simulink library "cntrl_atti_red_indi_lib"  (R2018b)
settings: Solver=VariableStepAuto  StartTime=0.0  StopTime=10.0  RelTol=1e-3
undefined symbols (not defined in the file or in its folder): atti_cntrl, DiscIntNeverNeededParam
libraries: angles_lib x3, ndi_lib x2, $bdroot x2, axes_transformation_lib x1
settings Model: Creator=Ybeyer  LastModifiedBy=Yannic
settings SFSimCC: SimUseLocalCustomCode=off
settings RTWCC: RTWUseLocalCustomCode=off
settings CodeAppCC: StateflowObjectComments=on

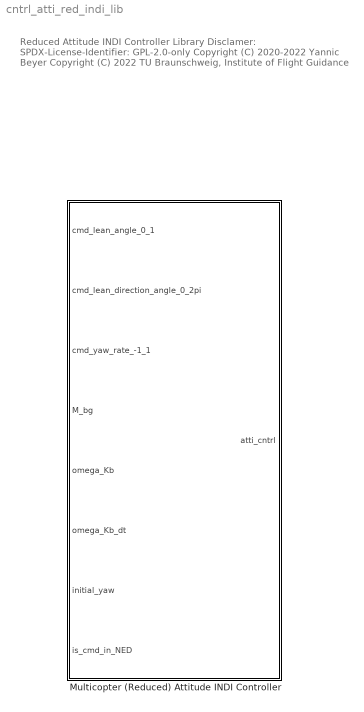
== system cntrl_atti_red_indi_lib ==
  note: Reduced Attitude INDI Controller Library
      |
      | Disclamer:
      | SPDX-License-Identifier: GPL-2.0-only
      |
      | Copyright (C) 2020-2022 Yannic Beyer
      | Copyright (C) 2022 TU Braunschweig, Institute of Flight Guidance
  Multicopter (Reduced) Attitude INDI Controller : Subsystem  mask{atti_cntrl=atti_cntrl, T=0.01}
      mask prompts: atti_cntrl "reduced attitude control struct"; T "inner loop time constant"
      mask Help: https://www.mathworks.com
      mask DialogControl DescGroupVar Prompt: INDI Reduced Attitude Controller
      mask DialogControl DescTextVar Prompt: To initialize the reduced attitude control struct see cntrlAttiRedIndiLoadParams

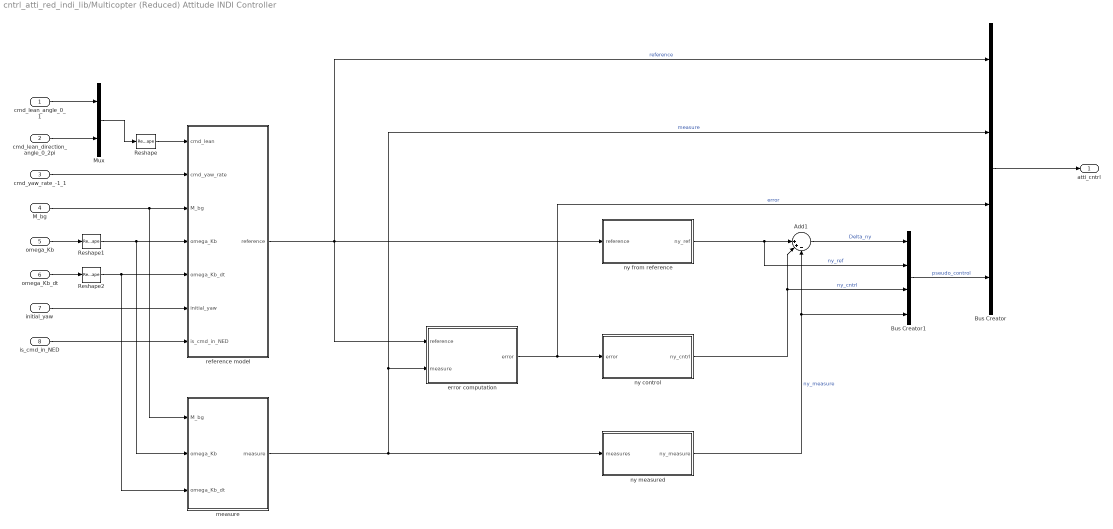
== system cntrl_atti_red_indi_lib/Multicopter (Reduced) Attitude INDI Controller ==
  cmd_lean_angle_0_1 : Inport
  cmd_lean_direction_angle_0_2pi : Inport  Port=2
  cmd_yaw_rate_-1_1 : Inport  Port=3
  M_bg : Inport  Port=4
  omega_Kb : Inport  Port=5
  omega_Kb_dt : Inport  Port=6
  initial_yaw : Inport  Port=7
  is_cmd_in_NED : Inport  Port=8
  Add1 : Sum  Inputs=||++-
  Bus Creator : BusCreator  Inputs=4
  Bus Creator1 : BusCreator  Inputs=4
  Mux : Mux  Inputs=2
  Reshape : Reshape  OutputDimensionality=Column vector (2-D)
  Reshape1 : Reshape  OutputDimensionality=Column vector (2-D)
  Reshape2 : Reshape  OutputDimensionality=Column vector (2-D)
  error computation : Subsystem
  measure : Subsystem
  ny control : Subsystem
  ny from reference : Subsystem
  ny measured : Subsystem
  reference model : Subsystem
  atti_cntrl : Outport
  wires:
  ny from reference/1(ny_ref) -> Bus Creator1/2, Add1/1  "ny_ref"
  Mux/1 -> Reshape/1
  error computation/1(error) -> ny control/1(error), Bus Creator/3  "error"
  omega_Kb_dt/1 -> Reshape2/1
  ny control/1(ny_cntrl) -> Bus Creator1/3, Add1/2  "ny_cntrl"
  ny measured/1(ny_measure) -> Bus Creator1/4, Add1/3  "ny_measure"
  reference model/1(reference) -> Bus Creator/1, error computation/1(reference), ny from reference/1(reference)  "reference"
  initial_yaw/1 -> reference model/6(initial_yaw)
  Bus Creator/1 -> atti_cntrl/1
  Bus Creator1/1 -> Bus Creator/4  "pseudo_control"
  Add1/1 -> Bus Creator1/1  "Delta_ny"
  M_bg/1 -> measure/1(M_bg), reference model/3(M_bg)
  omega_Kb/1 -> Reshape1/1
  measure/1(measure) -> Bus Creator/2, error computation/2(measure), ny measured/1(measures)  "measure"
  Reshape/1 -> reference model/1(cmd_lean)
  Reshape1/1 -> measure/2(omega_Kb), reference model/4(omega_Kb)
  Reshape2/1 -> measure/3(omega_Kb_dt), reference model/5(omega_Kb_dt)
  cmd_lean_angle_0_1/1 -> Mux/1
  cmd_lean_direction_angle_0_2pi/1 -> Mux/2
  cmd_yaw_rate_-1_1/1 -> reference model/2(cmd_yaw_rate)
  is_cmd_in_NED/1 -> reference model/7(is_cmd_in_NED)

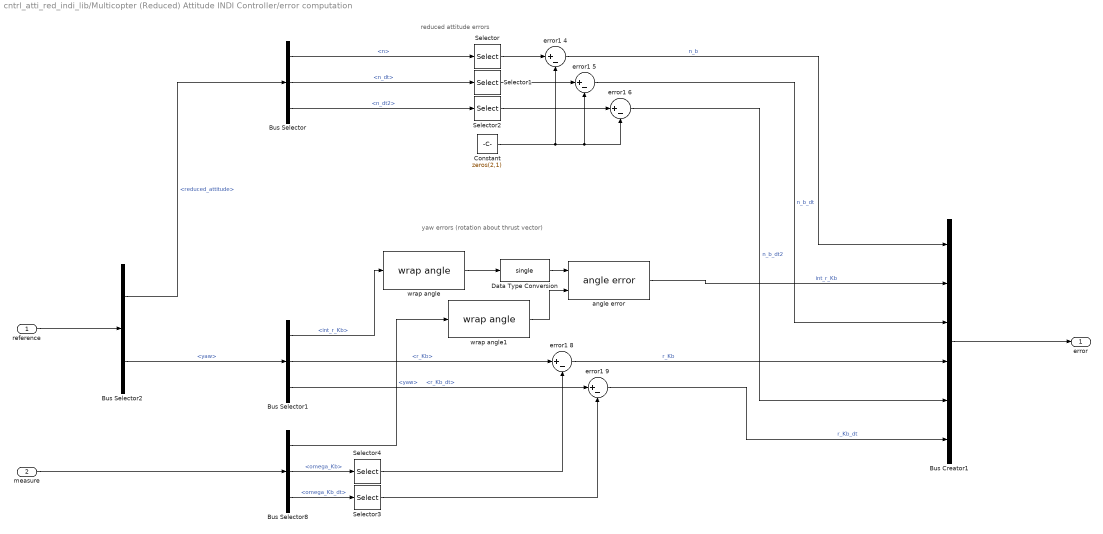
== system cntrl_atti_red_indi_lib/Multicopter (Reduced) Attitude INDI Controller/error computation ==
  note: reduced attitude errors
  note: yaw errors (rotation about thrust vector)
  reference : Inport
  measure : Inport  Port=2
  Bus Creator1 : BusCreator  Inputs=6
  Bus Selector : BusSelector  OutputSignals=n,n_dt,n_dt2
  Bus Selector1 : BusSelector  OutputSignals=int_r_Kb,r_Kb,r_Kb_dt
  Bus Selector2 : BusSelector  OutputSignals=reduced_attitude,yaw
  Bus Selector8 : BusSelector  OutputSignals=yaw,omega_Kb,omega_Kb_dt
  Constant : Constant  Value=zeros(2,1)  OutDataTypeStr=Inherit: Inherit via back propagation
  Data Type Conversion : DataTypeConversion  OutDataTypeStr=single
  Selector : Selector  InputPortWidth=3  IndexOptions=Index vector (dialog)  Indices=[1,2]  OutputSizes=1
  Selector1 : Selector  InputPortWidth=3  IndexOptions=Index vector (dialog)  Indices=[1,2]  OutputSizes=1
  Selector2 : Selector  InputPortWidth=3  IndexOptions=Index vector (dialog)  Indices=[1,2]  OutputSizes=1
  Selector3 : Selector  InputPortWidth=3  IndexOptions=Index vector (dialog)  Indices=3  OutputSizes=1
  Selector4 : Selector  InputPortWidth=3  IndexOptions=Index vector (dialog)  Indices=3  OutputSizes=1
  angle error : angles_lib/angle error  SystemSampleTime=-1
      settings: SourceProductName=LADAC
  error1 {4..6,8..9} (5 alike) : Sum  Inputs=|+-
  wrap angle : angles_lib/wrap angle  SystemSampleTime=-1
      settings: SourceProductName=LADAC
  wrap angle1 : angles_lib/wrap angle  SystemSampleTime=-1
      settings: SourceProductName=LADAC
  error : Outport
  wires:
  error1 4/1 -> Bus Creator1/1  "n_b"
  reference/1 -> Bus Selector2/1
  Bus Selector/1 -> Selector/1  "<n>"
  Bus Selector/2 -> Selector1/1  "<n_dt>"
  Bus Selector/3 -> Selector2/1  "<n_dt2>"
  Bus Selector2/1 -> Bus Selector/1  "<reduced_attitude>"
  Bus Creator1/1 -> error/1
  Selector/1 -> error1 4/1
  Selector1/1 -> error1 5/1
  Selector2/1 -> error1 6/1
  Constant/1 -> error1 6/2, error1 5/2, error1 4/2
  Bus Selector2/2 -> Bus Selector1/1  "<yaw>"
  Bus Selector1/1 -> wrap angle/1  "<int_r_Kb>"
  Bus Selector1/2 -> error1 8/1  "<r_Kb>"
  Bus Selector1/3 -> error1 9/1  "<r_Kb_dt>"
  measure/1 -> Bus Selector8/1
  Bus Selector8/3 -> Selector3/1  "<omega_Kb_dt>"
  Bus Selector8/2 -> Selector4/1  "<omega_Kb>"
  Bus Selector8/1 -> wrap angle1/1  "<yaw>"
  Selector4/1 -> error1 8/2
  Selector3/1 -> error1 9/2
  angle error/1 -> Bus Creator1/2  "int_r_Kb"
  error1 8/1 -> Bus Creator1/4  "r_Kb"
  error1 5/1 -> Bus Creator1/3  "n_b_dt"
  error1 6/1 -> Bus Creator1/5  "n_b_dt2"
  error1 9/1 -> Bus Creator1/6  "r_Kb_dt"
  wrap angle1/1 -> angle error/2
  wrap angle/1 -> Data Type Conversion/1
  Data Type Conversion/1 -> angle error/1

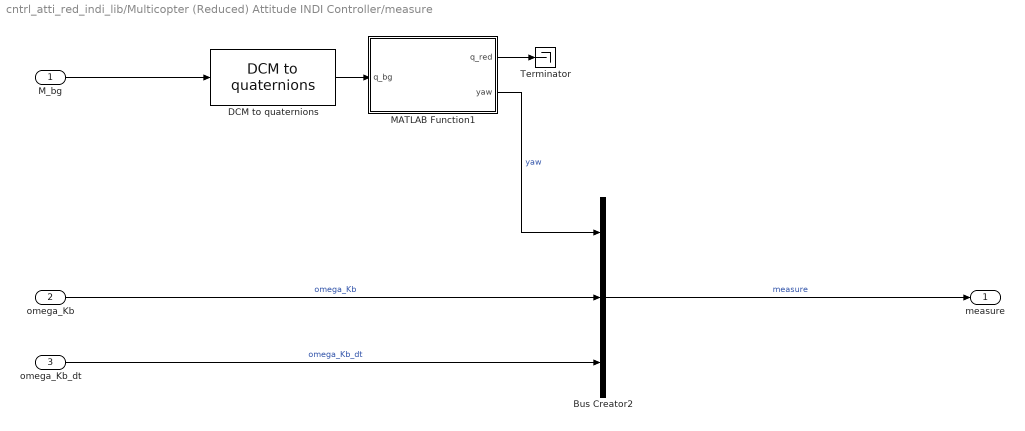
== system cntrl_atti_red_indi_lib/Multicopter (Reduced) Attitude INDI Controller/measure ==
  M_bg : Inport
  omega_Kb : Inport  Port=2
  omega_Kb_dt : Inport  Port=3
  Bus Creator2 : BusCreator  Inputs=3
  DCM to quaternions : axes_transformation_lib/DCM to quaternions  SystemSampleTime=-1
  MATLAB Function1 : MATLAB Function  TreatAsAtomicUnit=on
  Terminator : Terminator
  measure : Outport
  wires:
  DCM to quaternions/1 -> MATLAB Function1/1(q_bg)
  MATLAB Function1/1(q_red) -> Terminator/1
  MATLAB Function1/2(yaw) -> Bus Creator2/1  "yaw"
  M_bg/1 -> DCM to quaternions/1
  omega_Kb/1 -> Bus Creator2/2  "omega_Kb"
  omega_Kb_dt/1 -> Bus Creator2/3  "omega_Kb_dt"
  Bus Creator2/1 -> measure/1  "measure"

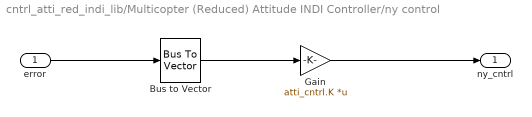
== system cntrl_atti_red_indi_lib/Multicopter (Reduced) Attitude INDI Controller/ny control ==
  error : Inport
  Bus to Vector : BusToVector
  Gain : Gain  Gain=atti_cntrl.K  Multiplication=Matrix(K*u)
  ny_cntrl : Outport
  wires:
  Gain/1 -> ny_cntrl/1
  error/1 -> Bus to Vector/1
  Bus to Vector/1 -> Gain/1

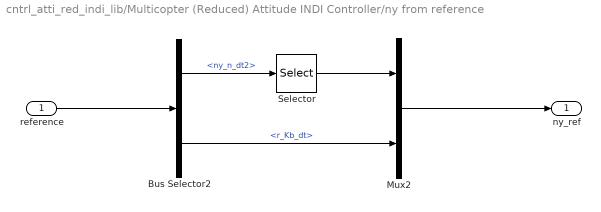
== system cntrl_atti_red_indi_lib/Multicopter (Reduced) Attitude INDI Controller/ny from reference ==
  reference : Inport
  Bus Selector2 : BusSelector  OutputSignals=reduced_attitude.ny_n_dt2,yaw.r_Kb_dt
  Mux2 : Mux  Inputs=2
  Selector : Selector  InputPortWidth=3  IndexOptions=Index vector (dialog)  Indices=[1,2]  OutputSizes=1
  ny_ref : Outport
  wires:
  reference/1 -> Bus Selector2/1
  Mux2/1 -> ny_ref/1
  Bus Selector2/2 -> Mux2/2  "<r_Kb_dt>"
  Bus Selector2/1 -> Selector/1  "<ny_n_dt2>"
  Selector/1 -> Mux2/1

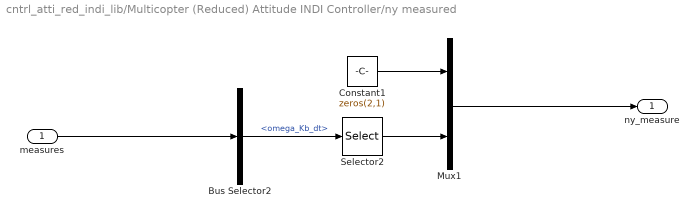
== system cntrl_atti_red_indi_lib/Multicopter (Reduced) Attitude INDI Controller/ny measured ==
  measures : Inport
  Bus Selector2 : BusSelector  OutputSignals=attitude.omega_Kb_dt
  Constant1 : Constant  Value=zeros(2,1)  OutDataTypeStr=Inherit: Inherit via back propagation
  Mux1 : Mux  Inputs=2
  Selector2 : Selector  InputPortWidth=3  IndexOptions=Index vector (dialog)  Indices=3  OutputSizes=1
  ny_measure : Outport
  wires:
  Bus Selector2/1 -> Selector2/1  "<omega_Kb_dt>"
  measures/1 -> Bus Selector2/1
  Mux1/1 -> ny_measure/1
  Selector2/1 -> Mux1/2
  Constant1/1 -> Mux1/1

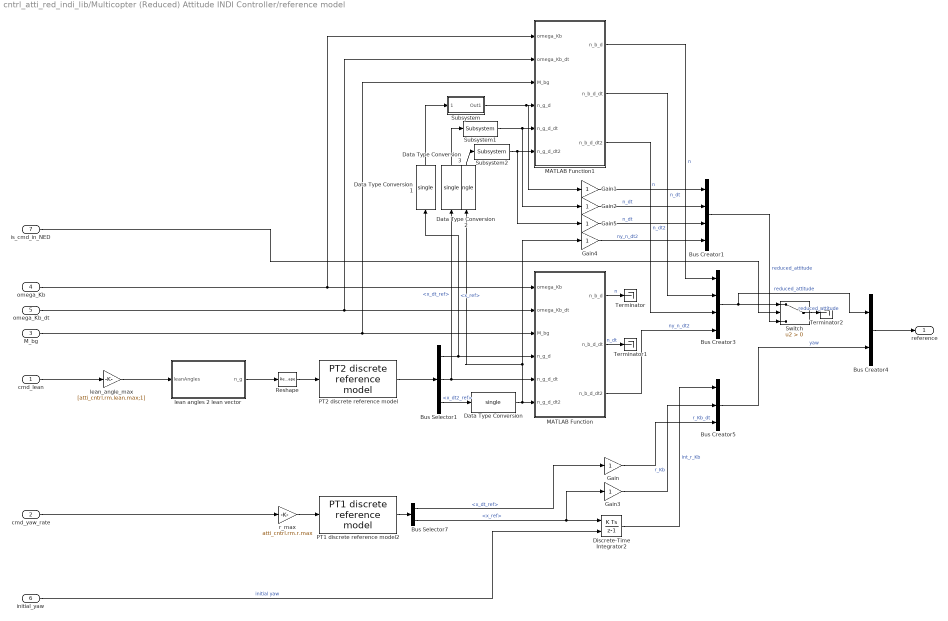
== system cntrl_atti_red_indi_lib/Multicopter (Reduced) Attitude INDI Controller/reference model ==
  cmd_lean : Inport
  cmd_yaw_rate : Inport  Port=2
  M_bg : Inport  Port=3
  omega_Kb : Inport  Port=4
  omega_Kb_dt : Inport  Port=5
  initial_yaw : Inport  Port=6
  is_cmd_in_NED : Inport  Port=7
  Bus Creator1 : BusCreator  Inputs=4
  Bus Creator3 : BusCreator  Inputs=4
  Bus Creator4 : BusCreator  Inputs=2
  Bus Creator5 : BusCreator  Inputs=3
  Bus Selector1 : BusSelector  OutputSignals=x_ref,x_dt_ref,x_dt2_ref
  Bus Selector7 : BusSelector  OutputSignals=x_dt_ref,x_ref
  Data Type Conversion{,1..3} (4 alike) : DataTypeConversion  OutDataTypeStr=single
  Discrete-Time Integrator2 : DiscreteIntegrator  InitialConditionSource=external  SampleTime=-1  ICPrevOutput=DiscIntNeverNeededParam  ICPrevScaledInput=DiscIntNeverNeededParam
  Gain{,1..5} (6 alike) : Gain
  MATLAB Function : MATLAB Function  TreatAsAtomicUnit=on
  MATLAB Function1 : MATLAB Function  TreatAsAtomicUnit=on
  PT1 discrete reference model2 : ndi_lib/PT1 discrete reference model  T=atti_cntrl.rm.r.T  x_max=inf  x_min=-inf  x_dt_max=inf  x_dt_min=-inf  x_init=0
  PT2 discrete reference model : ndi_lib/PT2 discrete reference model  omega=atti_cntrl.rm.lean.omega  d=atti_cntrl.rm.lean.D  x_dt2_max=inf  x_dt2_min=-inf  x_dt_max=inf  x_dt_min=-inf  x_max=inf  x_min=-inf  x_init=single([0;0;-1])  x_dt_init=0
  Reshape : Reshape  OutputDimensionality=Column vector (2-D)
  Subsystem : Subsystem
  Subsystem1 : $bdroot/Multicopter (Reduced) Attitude INDI Controller/reference model/Subsystem  SystemSampleTime=-1
  Subsystem2 : $bdroot/Multicopter (Reduced) Attitude INDI Controller/reference model/Subsystem  SystemSampleTime=-1
  Switch : Switch  Criteria=u2 > Threshold
  Terminator : Terminator
  Terminator1 : Terminator
  Terminator2 : Terminator
  lean angles 2 lean vector : MATLAB Function  TreatAsAtomicUnit=on
  lean_angle_max : Gain  Gain=[atti_cntrl.rm.lean.max;1]
  r_max : Gain  Gain=atti_cntrl.rm.r.max
  reference : Outport
  wires:
  initial_yaw/1 -> Discrete-Time Integrator2/2  "initial yaw"
  Bus Selector1/1 -> Data Type Conversion1/1, MATLAB Function/4(n_g_d)  "<x_ref>"
  MATLAB Function/3(n_b_d_dt2) -> Bus Creator3/4  "ny_n_dt2"
  PT2 discrete reference model/1 -> Bus Selector1/1
  MATLAB Function1/2(n_b_d_dt) -> Bus Creator3/2  "n_dt"
  Bus Selector1/2 -> MATLAB Function/5(n_g_d_dt), Data Type Conversion3/1  "<x_dt_ref>"
  Bus Selector1/3 -> Data Type Conversion/1  "<x_dt2_ref>"
  MATLAB Function1/1(n_b_d) -> Bus Creator3/1  "n"
  lean angles 2 lean vector/1(n_g) -> Reshape/1
  Bus Creator4/1 -> reference/1
  Bus Creator3/1 -> Bus Creator4/1, Switch/1  "reduced_attitude"
  omega_Kb/1 -> MATLAB Function1/1(omega_Kb), MATLAB Function/1(omega_Kb)
  omega_Kb_dt/1 -> MATLAB Function1/2(omega_Kb_dt), MATLAB Function/2(omega_Kb_dt)
  M_bg/1 -> MATLAB Function1/3(M_bg), MATLAB Function/3(M_bg)
  cmd_yaw_rate/1 -> r_max/1
  r_max/1 -> PT1 discrete reference model2/1
  Bus Selector7/1 -> Gain/1  "<x_dt_ref>"
  PT1 discrete reference model2/1 -> Bus Selector7/1
  Bus Selector7/2 -> Gain3/1, Discrete-Time Integrator2/1  "<x_ref>"
  Bus Creator5/1 -> Bus Creator4/2  "yaw"
  Discrete-Time Integrator2/1 -> Bus Creator5/1  "int_r_Kb"
  Gain/1 -> Bus Creator5/3  "r_Kb_dt"
  Gain3/1 -> Bus Creator5/2  "r_Kb"
  Data Type Conversion/1 -> MATLAB Function/6(n_g_d_dt2), Gain4/1, Data Type Conversion2/1
  cmd_lean/1 -> lean_angle_max/1
  Reshape/1 -> PT2 discrete reference model/1
  Bus Creator1/1 -> Switch/3  "reduced_attitude"
  is_cmd_in_NED/1 -> Switch/2
  Gain1/1 -> Bus Creator1/1  "n"
  Gain2/1 -> Bus Creator1/2  "n_dt"
  Gain4/1 -> Bus Creator1/4  "ny_n_dt2"
  lean_angle_max/1 -> lean angles 2 lean vector/1(leanAngles)
  Data Type Conversion1/1 -> Subsystem/1(<x_ref>)
  Data Type Conversion3/1 -> Subsystem1/1
  Data Type Conversion2/1 -> Subsystem2/1
  MATLAB Function1/3(n_b_d_dt2) -> Bus Creator3/3  "n_dt2"
  MATLAB Function/1(n_b_d) -> Terminator/1  "n"
  MATLAB Function/2(n_b_d_dt) -> Terminator1/1  "n_dt"
  Gain5/1 -> Bus Creator1/3  "n_dt"
  Switch/1 -> Terminator2/1  "reduced_attitude"
  Subsystem/1(Out1) -> Gain1/1, MATLAB Function1/4(n_g_d)
  Subsystem1/1 -> MATLAB Function1/5(n_g_d_dt), Gain2/1
  Subsystem2/1 -> Gain5/1, MATLAB Function1/6(n_g_d_dt2)

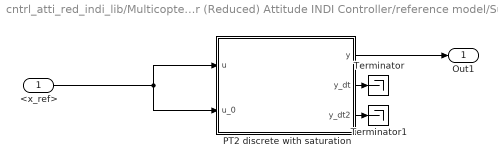
== system cntrl_atti_red_indi_lib/Multicopter (Reduced) Attitude INDI Controller/reference model/Subsystem ==
  <x_ref> : Inport
  PT2 discrete with saturation : Subsystem  mask{omega=2./T, d=1, x_dt2_max=inf, x_dt2_min=-inf, x_dt_max=inf, x_dt_min=-inf, x_max=inf, x_min=-inf, x_init=0, x_dt_init=0}
      mask prompts: omega "Natural frequency"; d "Damping ratio"; x_dt2_max "Maximum acceleration"; x_dt2_min "Minimum acceleration"; x_dt_max "Maximum rate"; x_dt_min "Minimum rate"; x_max "Maximum position"; x_min "Minimum position"; x_init "Initial position"; x_dt_init "Initial rate"
  Terminator : Terminator
  Terminator1 : Terminator
  Out1 : Outport
  wires:
  PT2 discrete with saturation/2(y_dt) -> Terminator/1
  PT2 discrete with saturation/3(y_dt2) -> Terminator1/1
  PT2 discrete with saturation/1(y) -> Out1/1
  <x_ref>/1 -> PT2 discrete with saturation/2(u_0), PT2 discrete with saturation/1(u)

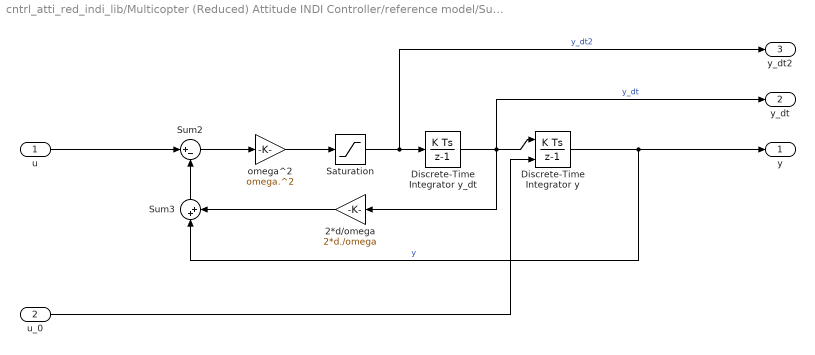
== system cntrl_atti_red_indi_lib/Multicopter (Reduced) Attitude INDI Controller/reference model/Subsystem/PT2 discrete with saturation ==
  u : Inport
  u_0 : Inport  Port=2
  2*d/omega : Gain  Gain=2*d./omega
  Discrete-Time Integrator y : DiscreteIntegrator  InitialConditionSource=external  InitialCondition=x_init  SampleTime=-1  OutDataTypeStr=Inherit: Inherit via back propagation  LimitOutput=on  UpperSaturationLimit=x_max  LowerSaturationLimit=x_min  ICPrevOutput=DiscIntNeverNeededParam  ICPrevScaledInput=DiscIntNeverNeededParam
  Discrete-Time Integrator y_dt : DiscreteIntegrator  InitialCondition=x_dt_init  SampleTime=-1  OutDataTypeStr=Inherit: Inherit via back propagation  LimitOutput=on  UpperSaturationLimit=x_dt_max  LowerSaturationLimit=x_dt_min  ICPrevOutput=DiscIntNeverNeededParam  ICPrevScaledInput=DiscIntNeverNeededParam
  Saturation : Saturate  UpperLimit=x_dt2_max  LowerLimit=x_dt2_min
  Sum2 : Sum  Inputs=|+-
  Sum3 : Sum  Inputs=|++
  omega^2 : Gain  Gain=omega.^2
  y : Outport
  y_dt : Outport  Port=2
  y_dt2 : Outport  Port=3
  wires:
  Saturation/1 -> y_dt2/1, Discrete-Time Integrator y_dt/1  "y_dt2"
  omega^2/1 -> Saturation/1
  Sum3/1 -> Sum2/2
  u/1 -> Sum2/1
  2*d/omega/1 -> Sum3/2
  Sum2/1 -> omega^2/1
  Discrete-Time Integrator y/1 -> Sum3/1, y/1  "y"
  Discrete-Time Integrator y_dt/1 -> 2*d/omega/1, y_dt/1, Discrete-Time Integrator y/1  "y_dt"
  u_0/1 -> Discrete-Time Integrator y/2

== matlab function cntrl_atti_red_indi_lib/Multicopter (Reduced) Attitude INDI Controller/reference model/MATLAB Function ==
  data: n_b_d output; n_b_d_dt output; omega_Kb input; n_b_d_dt2 output; omega_Kb_dt input; M_bg input; n_g_d input; n_g_d_dt input; n_g_d_dt2 input
function [ n_b_d, n_b_d_dt, n_b_d_dt2]   = fcn(omega_Kb, omega_Kb_dt, M_bg, n_g_d, n_g_d_dt, n_g_d_dt2 )
% https://arxiv.org/pdf/2002.07837.pdf

% time derivative of rotation matrix
M_bg_dt = dcmDerivFromOmega( M_bg', omega_Kb )';

n_b_d = M_bg*n_g_d;

n_b = single([0;0;-1]);
rho = acos( max( -1, min( 1, dot( n_b_d, n_b ) ) ) );

% eq. (7)
n_b_d_dt = -cross(omega_Kb,n_b_d) + M_bg*n_g_d_dt;

% time derivative of eq. (7)
n_b_d_dt2 = -cross(omega_Kb_dt,n_b_d) -cross(omega_Kb,n_b_d_dt) ...
    + M_bg_dt*n_g_d_dt + M_bg*n_g_d_dt2;

% manipulate desired vector if it is tilted more than 90 degrees
if n_b_d(3) > 0
    n_b_d(3) = 0;
    %n_b_d = n_b_d/(eps(n_b_d(1))+norm(n_b_d,2));
    % increase h1 and h2 up to 2 (2 for 180 degrees)
    n_b_d(1:2) = n_b_d(1:2) + 2*( n_b_d(1:2)/(eps(n_b_d(1))+norm(n_b_d(1:2),2)) - n_b_d(1:2) );
    if norm(n_b_d,2) < 0.9
        n_b_d(1) = -1;
        n_b_d = n_b_d/norm(n_b_d,2);
    end
    % sign must be flipped but it yields better results if the magnitude is
    % reduced
    n_b_d_dt = -n_b_d_dt*0.2;
    n_b_d_dt2 = -n_b_d_dt2*0.2;
end

end

== matlab function cntrl_atti_red_indi_lib/Multicopter (Reduced) Attitude INDI Controller/reference model/MATLAB Function1 ==
  data: n_b_d output; n_b_d_dt output; omega_Kb input; n_b_d_dt2 output; omega_Kb_dt input; M_bg input; n_g_d input; n_g_d_dt input; n_g_d_dt2 input
function [ n_b_d, n_b_d_dt, n_b_d_dt2]   = fcn(omega_Kb, omega_Kb_dt, M_bg, n_g_d, n_g_d_dt, n_g_d_dt2 )
% https://arxiv.org/pdf/2002.07837.pdf

% time derivative of rotation matrix
M_bg_dt = dcmDerivFromOmega( M_bg', omega_Kb )';

n_b_d = M_bg*n_g_d;

n_b = single([0;0;-1]);
rho = acos( max( -1, min( 1, dot( n_b_d, n_b ) ) ) );

% eq. (7)
n_b_d_dt = -cross(omega_Kb,n_b_d) + M_bg*n_g_d_dt;

% time derivative of eq. (7)
n_b_d_dt2 = -cross(omega_Kb_dt,n_b_d) -cross(omega_Kb,n_b_d_dt) ...
    + M_bg_dt*n_g_d_dt + M_bg*n_g_d_dt2;

% manipulate desired vector if it is tilted more than 90 degrees
if n_b_d(3) > 0
    n_b_d(3) = 0;
    %n_b_d = n_b_d/(eps(n_b_d(1))+norm(n_b_d,2));
    % increase h1 and h2 up to 2 (2 for 180 degrees)
    n_b_d(1:2) = n_b_d(1:2) + 2*( n_b_d(1:2)/(eps(n_b_d(1))+norm(n_b_d(1:2),2)) - n_b_d(1:2) );
    if norm(n_b_d,2) < 0.9
        n_b_d(1) = -1;
        n_b_d = n_b_d/norm(n_b_d,2);
    end
    % sign must be flipped but it yields better results if the magnitude is
    % reduced
    n_b_d_dt = -n_b_d_dt*0.2;
    n_b_d_dt2 = -n_b_d_dt2*0.2;
end

end

== matlab function cntrl_atti_red_indi_lib/Multicopter (Reduced) Attitude INDI Controller/reference model/lean angles 2 lean vector ==
  data: leanAngles input; n_g output
function n_g = leanAngles2leanVector( leanAngles )
n_g = leanAngles2leanVector( leanAngles );
end

== matlab function cntrl_atti_red_indi_lib/Multicopter (Reduced) Attitude INDI Controller/measure/MATLAB Function1 ==
  data: q_bg input; q_red output; yaw output
function [q_red,yaw] = fcn(q_bg)
[q_red,yaw] = quatReduced(q_bg);
end
